simulink model "control_block"  (R2023b)
settings: Solver=VariableStepAuto  StartTime=0.0  StopTime=30  RelTol=1e-3
settings Model: Creator=dee5127@AD.PSU.EDU  LastModifiedBy=ratne
settings SolverCC: AlgebraicLoopSolver=TrustRegion
settings DebuggingCC: ArithmeticOperatorsInVariantConditions=warning
settings SFSimCC: CustomCodeUndefinedFunction=UseInterfaceOnly
settings RTWCC: DLArmComputeVersion=19.05

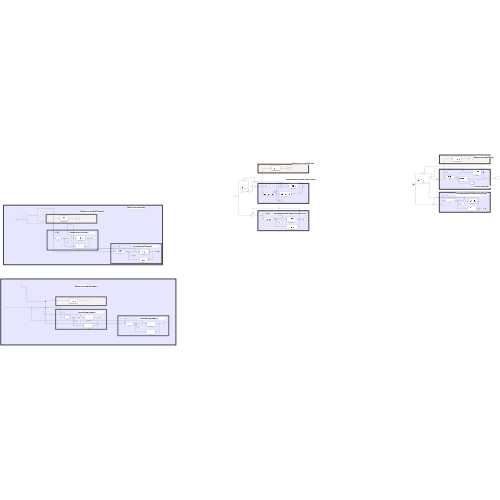
[thumbnail: Simulink's stored preview of the top-level diagram]
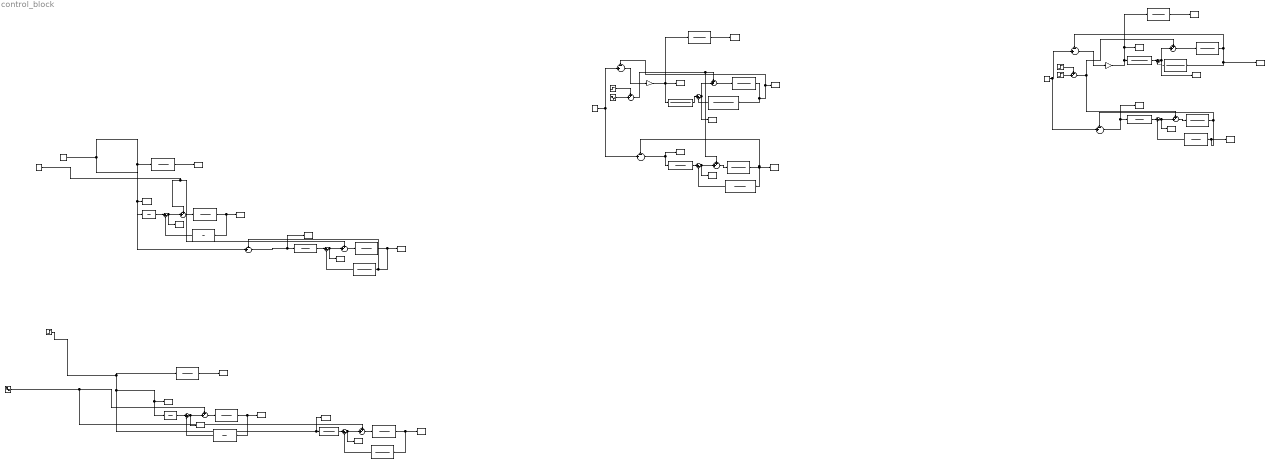
== system control_block ==
  note: Reference model(Rudder)
  note: U
  note: closed-loop(rudder)
  note: Reference model(Thruster)
  note: U
  note: closed-loop(Thruster)
  note: U
  note: closed-loop(rudder)
  note: U
  note: closed-loop(Thruster)
  note: Closed-loop(Yaw)
  note: Reference model(Yaw)
  note: compensated closed-loop(Thrust)
  note: Reference model(Thrust)
  note: uncompensated closed-loop(Thrust)
  note: U
  note: Not in use currently
  note: Uncompensated Closed-loop(Yaw)
  note: U
  Constant : Constant  Value=60
  Constant1 : Constant
  Constant2 : Constant
  Constant3 : Constant  Value=10
  Gain : Gain  Gain=4
  Gain1 : Gain  Gain=4
  Plant(Rudder) : TransferFcn  Numerator=[0.5 0]
  Plant(Rudder)1 : TransferFcn  Numerator=[0.5 0]
  Plant(Rudder)2 : TransferFcn  Numerator=[0.2 0.2]  Denominator=[1 0.5 0.8]
  Plant(Rudder)4 : TransferFcn  Numerator=[0.01 0.01]  Denominator=[1 0.2 0.1]
  Plant(Rudder)5 : TransferFcn  Numerator=[0.01 0.01]  Denominator=[1 0.2 0.1]
  Plant(Rudder)6 : TransferFcn  Numerator=[0.2 0.2]  Denominator=[1 0.5 0.8]
  Plant(Thruster) : TransferFcn  Numerator=[1 0]  Denominator=[1 5 1]
  Plant(Thruster)1 : TransferFcn  Numerator=[1 0]  Denominator=[1 5 1]
  REFERENCE MODEL : TransferFcn  Numerator=[0.7]  Denominator=[1 4 1]
  REFERENCE MODEL1 : TransferFcn  Numerator=[0.7]  Denominator=[1 4 1]
  REFERENCE MODEL2 : TransferFcn  Numerator=[4]  Denominator=[1 1.4 1]
  REFERENCE MODEL3 : TransferFcn  Numerator=[10]  Denominator=[1 1.4 1]
  S/R1 : TransferFcn  Numerator=[2 0]  Denominator=[0.5 0]
  S/R2 : TransferFcn  Numerator=[-1 0]  Denominator=[1 0]
  S/R3 : TransferFcn  Numerator=[13 42 11]  Denominator=[0.5 -0.5 0]
  S/R4 : TransferFcn  Numerator=[10 45 11]  Denominator=[1 -1 0]
  S/R5 : TransferFcn  Numerator=[8.9 4.83 7.8]  Denominator=[0.2 0.6 0.4]
  S/R6 : TransferFcn  Numerator="[9.2 10.9  7.1]"  Denominator=[0.01 0.03 0.02]
  S/R7 : TransferFcn  Numerator=[1.2 0.9]  Denominator=[0.01 0.01]
  S/R8 : TransferFcn  Numerator=[0.9 0.2]  Denominator=[0.2 0.2]
  Sine Wave : Sin  SampleTime=0
  Sine Wave1 : Sin  SampleTime=0
  Step1 : Step  After=25  SampleTime=0
  Step4 : Step  After=4  SampleTime=0
  Step5 : Step  After=3  SampleTime=0
  Step8 : Step  After=4  SampleTime=0
  Sum{1,3,5,7,10,14,18,21} (8 alike) : Sum  Inputs=|+-
  Sum{2,4,6,8,11,13,15,17,19,22} (10 alike) : Sum  Inputs=+|+||
  Sum{9,12,16,20,23} (5 alike) : Sum  Inputs=-|+||
  T/R1 : TransferFcn  Numerator=[0.7]  Denominator=[0.5 0]
  T/R2 : TransferFcn  Numerator=[0.7]  Denominator=[1 0]
  T/R3 : TransferFcn  Numerator=[0.7 7]  Denominator=[0.5 -0.5 0]
  T/R4 : TransferFcn  Numerator=[0.7 0.7]  Denominator=[4 -4 0]
  T/R5 : TransferFcn  Numerator=[28 37.8]  Denominator=[0.2 0.6 0.4]
  T/R6 : TransferFcn  Numerator=[10.5 73.5]  Denominator=[0.01 0.03 0.02]
  T/R7 : TransferFcn  Numerator=[10]  Denominator=[0.01 0.01]
  T/R8 : TransferFcn  Numerator=[4]  Denominator=[0.2 0.2]
  To Workspace1 : ToWorkspace  VariableName=Ym1  SampleTime=-1
  To Workspace10 : ToWorkspace  VariableName=uc2  SampleTime=-1
  To Workspace11 : ToWorkspace  VariableName=U  SampleTime=-1
  To Workspace12 : ToWorkspace  VariableName=Y3  SampleTime=-1
  To Workspace13 : ToWorkspace  VariableName=uc3  SampleTime=-1
  To Workspace14 : ToWorkspace  VariableName=U3  SampleTime=-1
  To Workspace15 : ToWorkspace  VariableName=uc4  SampleTime=-1
  To Workspace16 : ToWorkspace  VariableName=U4  SampleTime=-1
  To Workspace17 : ToWorkspace  VariableName=Y4  SampleTime=-1
  To Workspace18 : ToWorkspace  VariableName=Ym2  SampleTime=-1
  To Workspace19 : ToWorkspace  VariableName=uc5  SampleTime=-1
  To Workspace2 : ToWorkspace  VariableName=Y2  SampleTime=-1
  To Workspace20 : ToWorkspace  VariableName=U5  SampleTime=-1
  To Workspace21 : ToWorkspace  VariableName=Y5  SampleTime=-1
  To Workspace22 : ToWorkspace  VariableName=Ym3  SampleTime=-1
  To Workspace23 : ToWorkspace  VariableName=uc6  SampleTime=-1
  To Workspace24 : ToWorkspace  VariableName=U6  SampleTime=-1
  To Workspace25 : ToWorkspace  VariableName=Y6  SampleTime=-1
  To Workspace26 : ToWorkspace  VariableName=uc7  SampleTime=-1
  To Workspace27 : ToWorkspace  VariableName=U7  SampleTime=-1
  To Workspace28 : ToWorkspace  VariableName=Y7  SampleTime=-1
  To Workspace3 : ToWorkspace  VariableName=Ym  SampleTime=-1
  To Workspace4 : ToWorkspace  VariableName=uc  SampleTime=-1
  To Workspace5 : ToWorkspace  VariableName=Y1  SampleTime=-1
  To Workspace6 : ToWorkspace  VariableName=uc1  SampleTime=-1
  To Workspace7 : ToWorkspace  VariableName=U1  SampleTime=-1
  To Workspace8 : ToWorkspace  VariableName=U2  SampleTime=-1
  To Workspace9 : ToWorkspace  VariableName=Y  SampleTime=-1
  wires:
  REFERENCE MODEL/1 -> To Workspace3/1
  S/R1/1 -> Sum3/2
  T/R1/1 -> Sum3/1
  Plant(Rudder)/1 -> S/R1/1, To Workspace5/1
  Sum4/1 -> Plant(Rudder)/1
  Sum3/1 -> Sum4/2, To Workspace7/1
  S/R2/1 -> Sum1/2
  REFERENCE MODEL1/1 -> To Workspace1/1
  Sum1/1 -> Sum2/2, To Workspace8/1
  Plant(Thruster)/1 -> S/R2/1, To Workspace2/1
  Sum2/1 -> Plant(Thruster)/1
  T/R2/1 -> Sum1/1
  Step1/1 -> To Workspace10/1, T/R3/1, T/R1/1, To Workspace6/1, REFERENCE MODEL/1
  Sum5/1 -> Sum6/2, To Workspace11/1
  T/R3/1 -> Sum5/1
  S/R3/1 -> Sum5/2
  Sum6/1 -> Plant(Rudder)1/1
  Sine Wave/1 -> Sum4/1, Sum6/1
  Constant2/1 -> Sum8/1, Sum2/1
  Constant1/1 -> T/R2/1, REFERENCE MODEL1/1, Sum9/2, To Workspace4/1
  Sum8/1 -> Plant(Thruster)1/1
  Plant(Thruster)1/1 -> Sum9/1, S/R4/1, To Workspace12/1
  S/R4/1 -> Sum7/2
  Sum7/1 -> Sum8/2, To Workspace14/1
  T/R4/1 -> Sum7/1
  Sum9/1 -> To Workspace13/1, T/R4/1
  T/R5/1 -> Sum10/1
  Sum10/1 -> Sum11/2, To Workspace16/1
  Sum11/1 -> Plant(Rudder)2/1
  S/R5/1 -> Sum10/2
  REFERENCE MODEL2/1 -> To Workspace18/1
  Plant(Rudder)1/1 -> To Workspace9/1, S/R3/1
  Plant(Rudder)2/1 -> To Workspace17/1, S/R5/1, Sum12/1
  Sum12/1 -> Gain/1
  Step4/1 -> Sum13/1
  Step5/1 -> Sum13/2
  Sum13/1 -> Sum11/1, Sum22/1
  Gain/1 -> To Workspace15/1, REFERENCE MODEL2/1, T/R5/1
  Constant/1 -> Sum12/2, Sum23/2
  Gain1/1 -> REFERENCE MODEL3/1, To Workspace19/1, T/R6/1
  Step8/1 -> Sum17/1
  Sum17/1 -> Sum15/1, Sum19/1
  Plant(Rudder)4/1 -> Sum16/1, To Workspace21/1, S/R6/1
  REFERENCE MODEL3/1 -> To Workspace22/1
  S/R6/1 -> Sum14/2
  T/R6/1 -> Sum14/1
  Sum15/1 -> Plant(Rudder)4/1
  Sum16/1 -> Gain1/1
  Sum14/1 -> Sum15/2, To Workspace20/1
  Constant3/1 -> Sum20/2, Sum16/2
  Sine Wave1/1 -> Sum17/2
  Sum18/1 -> Sum19/2, To Workspace24/1
  S/R7/1 -> Sum18/2
  Plant(Rudder)5/1 -> To Workspace25/1, Sum20/1, S/R7/1
  Sum19/1 -> Plant(Rudder)5/1
  T/R7/1 -> Sum18/1
  Sum20/1 -> T/R7/1, To Workspace23/1
  Plant(Rudder)6/1 -> To Workspace28/1, S/R8/1, Sum23/1
  S/R8/1 -> Sum21/2
  T/R8/1 -> Sum21/1
  Sum22/1 -> Plant(Rudder)6/1
  Sum21/1 -> Sum22/2, To Workspace27/1
  Sum23/1 -> To Workspace26/1, T/R8/1
